simulink model "Problem_5"  (R2020a)
settings: Solver=VariableStepAuto  StartTime=0.0  StopTime=10.0  RelTol=1e-3
settings Model: Creator=Ganesh  LastModifiedBy=Ganesh

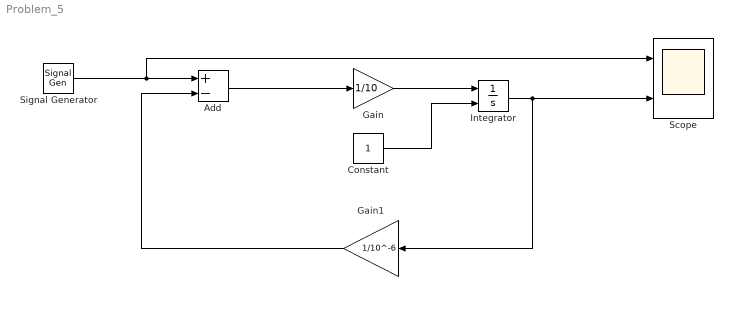
== system Problem_5 ==
  Add : Sum  Inputs=+-
  Constant : Constant
  Gain : Gain  Gain=1/10
  Gain1 : Gain  Gain=1/10^-6
  Integrator : Integrator  InitialConditionSource=external
  Scope : Scope  NumInputPorts=2
  Signal Generator : SignalGenerator  Units=rad/sec
  wires:
  Signal Generator/1 -> Scope/1, Add/1
  Add/1 -> Gain/1
  Gain1/1 -> Add/2
  Gain/1 -> Integrator/1
  Constant/1 -> Integrator/2
  Integrator/1 -> Gain1/1, Scope/2
